simulink model "DemoTR"  (R2022b)
settings: Solver=VariableStepAuto  StartTime=0.0  StopTime=10.0  RelTol=1e-3
libraries: ZLGUSBCAN x2
settings Model: Creator=admin  LastModifiedBy=admin

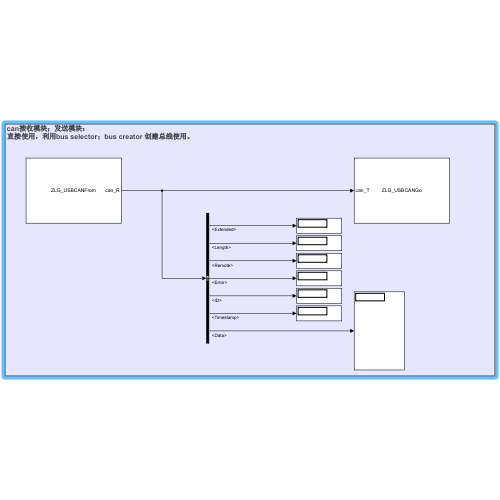
[thumbnail: Simulink's stored preview of the top-level diagram]
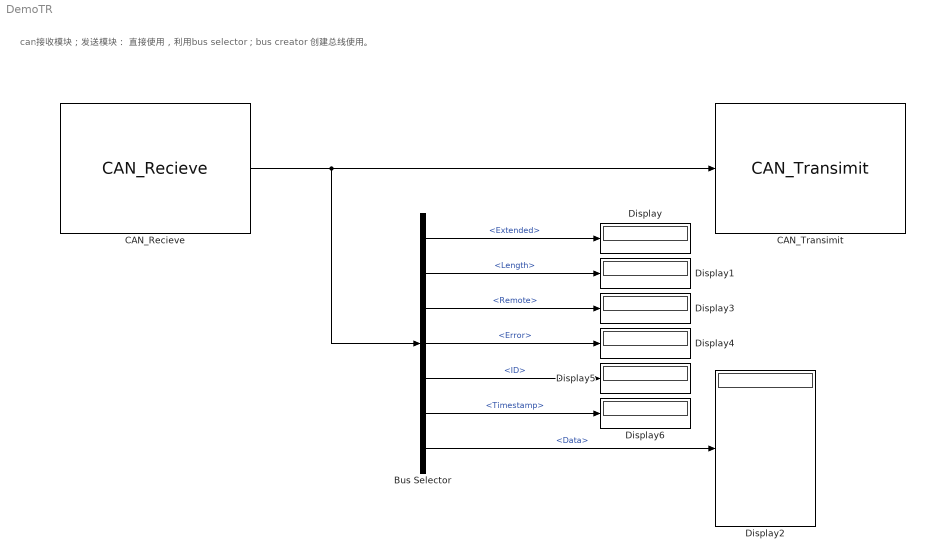
== system DemoTR ==
  note: can接收模块；发送模块：
      | 直接使用，利用bus selector；bus creator 创建总线使用。
  Bus Selector : BusSelector  OutputSignals=Extended,Length,Remote,Error,ID,Timestamp,Data
  CAN_Recieve : ZLGUSBCAN/CAN_Recieve  DeviceType=4  DeviceInd=0  ID=0x00000000  BaudRate=250
  CAN_Transimit : ZLGUSBCAN/CAN_Transimit  DeviceType=4  DeviceInd=0  ID=0x00000000  BaudRate=250
  Display{,1..6} (7 alike) : Display
      Display5 settings: Format=hex (Stored Integer)
  wires:
  CAN_Recieve/1 -> CAN_Transimit/1, Bus Selector/1
  Bus Selector/1 -> Display/1  "<Extended>"
  Bus Selector/2 -> Display1/1  "<Length>"
  Bus Selector/4 -> Display4/1  "<Error>"
  Bus Selector/5 -> Display5/1  "<ID>"
  Bus Selector/6 -> Display6/1  "<Timestamp>"
  Bus Selector/3 -> Display3/1  "<Remote>"
  Bus Selector/7 -> Display2/1  "<Data>"
